simulink model "Ex1"  (R2022b)
settings: Solver=VariableStepAuto  StartTime=0.0  StopTime=0.05  RelTol=1e-3
libraries: simulink x1, commrandsrc3 x1
settings Model: Creator=ASUS  LastModifiedBy=mluser
settings ModelReferenceCC: EnableRefExpFcnMdlSchedulingChecks=on

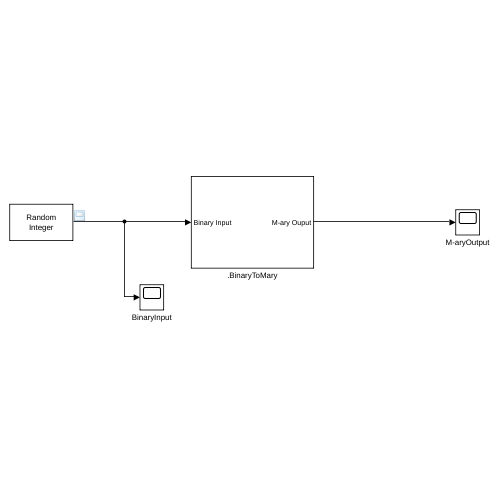
[thumbnail: Simulink's stored preview of the top-level diagram]
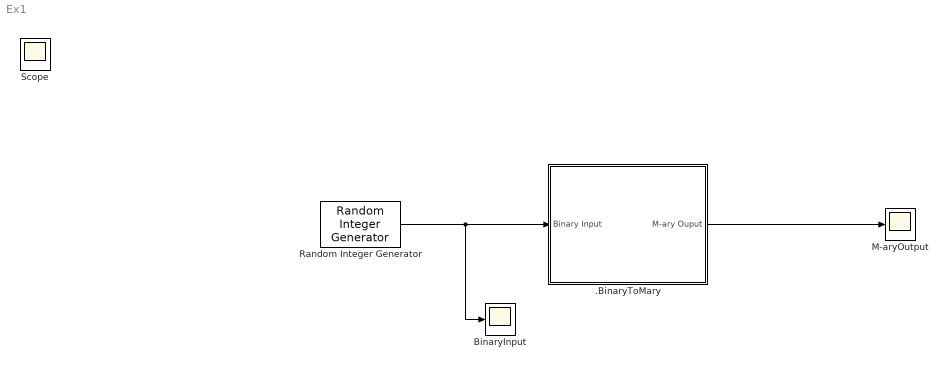
== system Ex1 ==
  .BinaryToMary : Subsystem
  BinaryInput : Scope
  M-aryOutput : Scope
  Random Integer Generator : commrandsrc3/Random Integer Generator  SetSize=2  SeedSource=Parameter  Seed=37  SampleTime=1e-3  SamplesPerFrame=1  OutputDataType=double  SimulateUsing=Interpreted execution
  Scope : Scope
  wires:
  .BinaryToMary/1(M-ary Ouput) -> M-aryOutput/1
  Random Integer Generator/1 -> BinaryInput/1, .BinaryToMary/1(Binary Input)

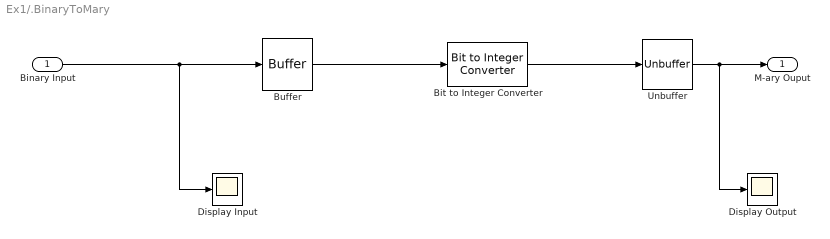
== system Ex1/.BinaryToMary ==
  Binary Input : Inport
  Bit to Integer Converter : simulink/Logic and Bit Operations/Bit to Integer Converter  nbits=3  bitOrder=MSB first  signedOutputValues=Unsigned  outDtype=Inherit via internal rule  outDtypeSigned=Inherit via internal rule
  Buffer : Buffer  N=3  OutputFrames=off
  Display Input : Scope
  Display Output : Scope
  Unbuffer : Unbuffer
  M-ary Ouput : Outport
  wires:
  Bit to Integer Converter/1 -> Unbuffer/1
  Unbuffer/1 -> Display Output/1, M-ary Ouput/1
  Buffer/1 -> Bit to Integer Converter/1
  Binary Input/1 -> Display Input/1, Buffer/1
